simulink model "car2"  (R2016a)
settings: Solver=VariableStepAuto  StartTime=0.0  StopTime=10.0  RelTol=1e-3
libraries: simulink x1
settings Model: Creator=richa  LastModifiedBy=richa

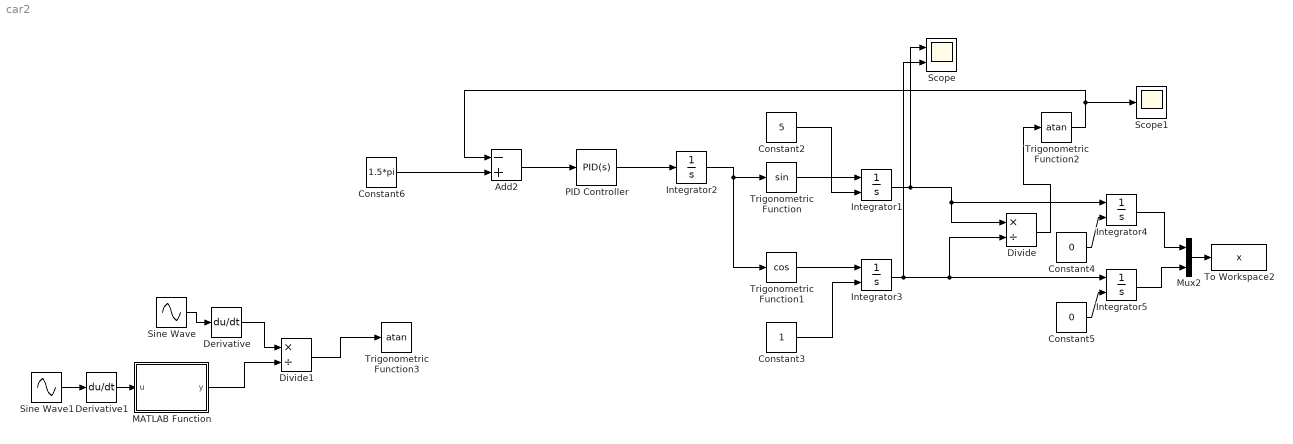
== system car2 ==
  Add2 : Sum  Inputs=-+
  Constant2 : Constant  Value=5
  Constant3 : Constant
  Constant4 : Constant  Value=0
  Constant5 : Constant  Value=0
  Constant6 : Constant  Value=1.5*pi
  Derivative : Derivative
  Derivative1 : Derivative
  Divide : Product  Inputs=*/
  Divide1 : Product  Inputs=*/
  Integrator{1,3..5} (4 alike) : Integrator  InitialConditionSource=external
  Integrator2 : Integrator
  MATLAB Function : MATLAB Function  TreatAsAtomicUnit=on
  Mux2 : Mux  Inputs=2
  PID Controller : simulink/Continuous/PID Controller  Controller=PID  TimeDomain=Continuous-time  SampleTime=-1  IntegratorMethod=Forward Euler  FilterMethod=Forward Euler  Form=Parallel  UseFilter=on  ControllerParametersSource=internal  P=0.1  I=0  D=0  N=100  InitialConditionSource=internal  InitialConditionForIntegrator=0  InitialConditionForFilter=0  ExternalReset=none  LimitOutput=off  UpperSaturationLimit=inf  LowerSaturationLimit=-inf  LinearizeAsGain=on  AntiWindupMode=none  Kb=1  TrackingMode=off  Kt=1  PParamMin=[]  PParamMax=[]  IParamMin=[]  IParamMax=[]  DParamMin=[]  DParamMax=[]  NParamMin=[]  NParamMax=[]  KbParamMin=[]  KbParamMax=[]  KtParamMin=[]  KtParamMax=[]  POutMin=[]  POutMax=[]  IOutMin=[]  IOutMax=[]  DOutMin=[]  DOutMax=[]  NOutMin=[]  NOutMax=[]  KbOutMin=[]  KbOutMax=[]  KtOutMin=[]  KtOutMax=[]  IntegratorOutMin=[]  IntegratorOutMax=[]  FilterOutMin=[]  FilterOutMax=[]  SumOutMin=[]  SumOutMax=[]  SumI1OutMin=[]  SumI1OutMax=[]  SumI2OutMin=[]  SumI2OutMax=[]  SumI3OutMin=[]  SumI3OutMax=[]  SumDOutMin=[]  SumDOutMax=[]  SaturationOutMin=[]  SaturationOutMax=[]  IntegratorContinuousStateAttributes=''  IntegratorStateMustResolveToSignalObject=off  IntegratorRTWStateStorageClass=Auto  FilterContinuousStateAttributes=''  FilterStateMustResolveToSignalObject=off  FilterRTWStateStorageClass=Auto  DifferentiatorICPrevScaledInput=0  DifferentiatorOutMin=[]  DifferentiatorOutMax=[]
  Scope : Scope  NumInputPorts=2
  Scope1 : Scope
  Sine Wave : Sin  Amplitude=100  SampleTime=0
  Sine Wave1 : Sin  Amplitude=100  Phase=pi/2  SampleTime=0
  To Workspace2 : ToWorkspace  VariableName=x  SampleTime=-1
  Trigonometric Function : Trigonometry
  Trigonometric Function1 : Trigonometry  Operator=cos
  Trigonometric Function2 : Trigonometry  Operator=atan
  Trigonometric Function3 : Trigonometry  Operator=atan
  wires:
  Add2/1 -> PID Controller/1
  PID Controller/1 -> Integrator2/1
  Integrator2/1 -> Trigonometric Function1/1, Trigonometric Function/1
  Divide/1 -> Trigonometric Function2/1
  Trigonometric Function2/1 -> Scope1/1, Add2/1
  Mux2/1 -> To Workspace2/1
  Trigonometric Function/1 -> Integrator1/1
  Integrator1/1 -> Scope/1, Integrator4/1, Divide/1
  Trigonometric Function1/1 -> Integrator3/1
  Integrator3/1 -> Integrator5/1, Divide/2, Scope/2
  Constant2/1 -> Integrator1/2
  Constant3/1 -> Integrator3/2
  Constant4/1 -> Integrator4/2
  Constant5/1 -> Integrator5/2
  Integrator4/1 -> Mux2/1
  Integrator5/1 -> Mux2/2
  Sine Wave/1 -> Derivative/1
  Sine Wave1/1 -> Derivative1/1
  Derivative/1 -> Divide1/1
  Divide1/1 -> Trigonometric Function3/1
  Derivative1/1 -> MATLAB Function/1(u)
  MATLAB Function/1(y) -> Divide1/2
  Constant6/1 -> Add2/2

== matlab function car2/MATLAB Function ==
  data: u input; y output
function y = fcn(u)
if(u<=0.001)
    y=0.001;
else
    y=u;
end

end
